simulink subsystem "LOGGING"  (R2025b)
settings: Solver=VariableStepAuto  StartTime=0.0  StopTime=10.0  RelTol=1e-3
settings Model: Creator=antoniohernandez-rodiciomateos  LastModifiedBy=antoniohernandez-rodiciomateos

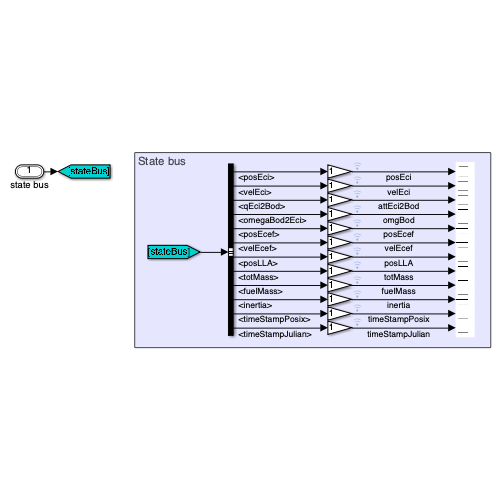
[thumbnail: Simulink's stored preview of the top-level diagram]
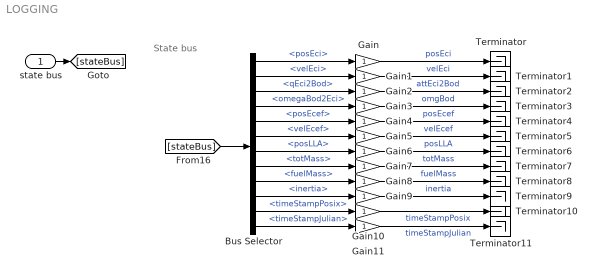
== system LOGGING ==
  note: State bus
  state bus : Inport  OutDataTypeStr=Bus: state_bus
  Bus Selector : BusSelector  OutputSignals=posEci,velEci,qEci2Bod,omegaBod2Eci,posEcef,velEcef,posLLA,totMass,fuelMass,inertia,timeStampPosix,timeStampJulian
  Gain{,1..11} (12 alike) : Gain
  Terminator{,1..11} (12 alike) : Terminator
  wires:
  state bus/1 -> [stateBus]
  [stateBus] -> Bus Selector/1
  Bus Selector/1 -> Gain/1  "<posEci>"
  Gain/1 -> Terminator/1  "posEci"
  Bus Selector/2 -> Gain1/1  "<velEci>"
  Gain1/1 -> Terminator1/1  "velEci"
  Gain3/1 -> Terminator3/1  "omgBod"
  Gain2/1 -> Terminator2/1  "attEci2Bod"
  Bus Selector/3 -> Gain2/1  "<qEci2Bod>"
  Bus Selector/4 -> Gain3/1  "<omegaBod2Eci>"
  Gain6/1 -> Terminator6/1  "posLLA"
  Gain7/1 -> Terminator7/1  "totMass"
  Gain5/1 -> Terminator5/1  "velEcef"
  Gain4/1 -> Terminator4/1  "posEcef"
  Bus Selector/5 -> Gain4/1  "<posEcef>"
  Bus Selector/6 -> Gain5/1  "<velEcef>"
  Bus Selector/7 -> Gain6/1  "<posLLA>"
  Bus Selector/8 -> Gain7/1  "<totMass>"
  Gain10/1 -> Terminator10/1  "timeStampPosix"
  Gain9/1 -> Terminator9/1  "inertia"
  Gain8/1 -> Terminator8/1  "fuelMass"
  Gain11/1 -> Terminator11/1  "timeStampJulian"
  Bus Selector/9 -> Gain8/1  "<fuelMass>"
  Bus Selector/10 -> Gain9/1  "<inertia>"
  Bus Selector/11 -> Gain10/1  "<timeStampPosix>"
  Bus Selector/12 -> Gain11/1  "<timeStampJulian>"
